simulink model "VOO_STATE"  (R2020a)
settings: Solver=FixedStepAuto  StartTime=0.0  StopTime=10.0  FixedStep=1e-3  RelTol=1e-3  EnableMultiTasking=on
undefined symbols (not defined in the file): D10, D12, D2, D5, D7, D9, PTA2, PTB9, PTC3, PTC4, PTD0, PTD3
libraries: frdmk64flib x8
settings Model: ExtModeTrigDuration=5  Creator=marry  LastModifiedBy=marry
settings OptimizationCC: EnhancedBackFolding=on  PassReuseOutputArgsAs=Individual arguments  ZeroExternalMemoryAtStartup=off  ZeroInternalMemoryAtStartup=off  MaxStackSize=64  OptimizeBlockOrder=speed  DifferentSizesBufferReuse=on  OptimizationCustomize=off  EfficientTunableParamExpr=on
settings DebuggingCC: ParameterTunabilityLossMsg=error
settings HardwareCC: ProdBitPerPointer=32  ProdBitPerSizeT=32  ProdBitPerPtrDiffT=32  ProdLargestAtomicInteger=Long  ProdLargestAtomicFloat=Double  ProdWordSize=32  ProdHWDeviceType=ARM Compatible->ARM Cortex
settings SFSimCC: MATLABDynamicMemAlloc=off
settings RTWCC: SystemTargetFile=ert.tlc  HardwareBoard=NXP FRDM-K64F  TemplateMakefile=ert_default_tmf  Toolchain=GNU Tools for ARM Embedded Processors
settings CodeAppCC: ForceParamTrailComments=on  IgnoreCustomStorageClasses=off  OperatorAnnotations=on  SimulinkDataObjDesc=on  SFDataObjDesc=on  InsertBlockDesc=on

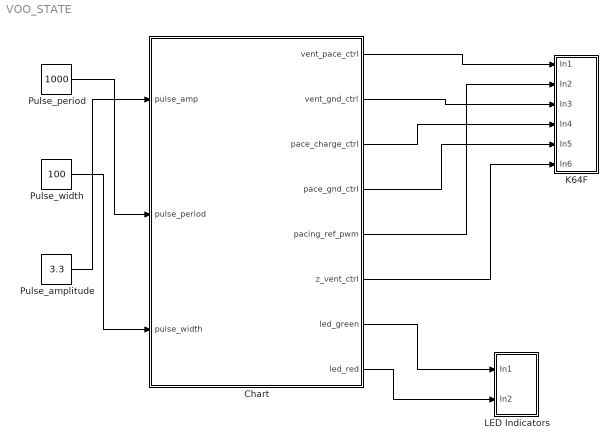
== system VOO_STATE ==
  Chart : Stateflow chart  TreatAsAtomicUnit=on
  K64F : Subsystem
  LED Indicators : Subsystem
  Pulse_amplitude : Constant  Value=3.3
  Pulse_period : Constant  Value=1000
  Pulse_width : Constant  Value=100
  wires:
  Chart/6(z_vent_ctrl) -> K64F/6(In6)
  Chart/4(pace_gnd_ctrl) -> K64F/5(In5)
  Chart/7(led_green) -> LED Indicators/1(In1)
  Chart/3(pace_charge_ctrl) -> K64F/4(In4)
  Chart/2(vent_gnd_ctrl) -> K64F/3(In3)
  Pulse_width/1 -> Chart/3(pulse_width)
  Chart/8(led_red) -> LED Indicators/2(In2)
  Pulse_amplitude/1 -> Chart/1(pulse_amp)
  Chart/1(vent_pace_ctrl) -> K64F/1(In1)
  Pulse_period/1 -> Chart/2(pulse_period)
  Chart/5(pacing_ref_pwm) -> K64F/2(In2)

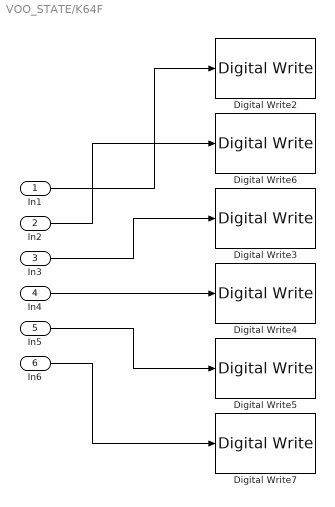
== system VOO_STATE/K64F ==
  In1 : Inport
  In2 : Inport  Port=2
  In3 : Inport  Port=3
  In4 : Inport  Port=4
  In5 : Inport  Port=5
  In6 : Inport  Port=6
  Digital Write2 : frdmk64flib/Digital Write  Whichpin=PTC4 (D9)
  Digital Write3 : frdmk64flib/Digital Write  Whichpin=PTD3 (D12)
  Digital Write4 : frdmk64flib/Digital Write  Whichpin=PTB9 (D2)
  Digital Write5 : frdmk64flib/Digital Write  Whichpin=PTD0 (D10)
  Digital Write6 : frdmk64flib/Digital Write  Whichpin=PTA2 (D5)
  Digital Write7 : frdmk64flib/Digital Write  Whichpin=PTC3 (D7)
  wires:
  In2/1 -> Digital Write6/1
  In1/1 -> Digital Write2/1
  In3/1 -> Digital Write3/1
  In4/1 -> Digital Write4/1
  In6/1 -> Digital Write7/1
  In5/1 -> Digital Write5/1

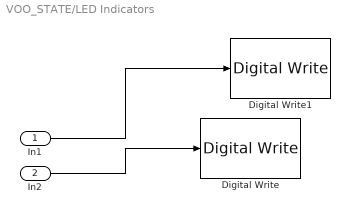
== system VOO_STATE/LED Indicators ==
  In1 : Inport
  In2 : Inport  Port=2
  Digital Write : frdmk64flib/Digital Write  Whichpin=RED_LED
  Digital Write1 : frdmk64flib/Digital Write  Whichpin=GREEN_LED
  wires:
  In1/1 -> Digital Write1/1
  In2/1 -> Digital Write/1

== stateflow chart VOO_STATE/Chart ==
  state AOO_Entry
    % Initial state when AOO is activated
    % Charging C22
    entry:
    vent_pace_ctrl = false;
    vent_gnd_ctrl = true;
    pace_charge_ctrl = true;
    pace_gnd_ctrl = true;
    pacing_ref_pwm = pulse_amp*20;
    z_vent_ctrl = 0;
    % LED indicator
    led_green = true;
    led_red = false;
  state AOO_Pace
    % Discharging current into the heart
    entry:
    pace_charge_ctrl = false;
    vent_gnd_ctrl = false;
    vent_pace_ctrl = true;
    % LED indicator
    led_green = false;
    led_red = true;
  state AOO_Charge
    % Charging C22 and C21 for cycles
    entry:
    vent_pace_ctrl = false;
    pace_charge_ctrl = true;
    vent_gnd_ctrl = true;
    % LED indicator
    led_green = true;
    led_red = false;
  (default) -> AOO_Entry
  AOO_Entry -> AOO_Pace : [after(pulse_period, msec)]
  AOO_Pace -> AOO_Charge : [after(pulse_width, msec)]
  AOO_Charge -> AOO_Pace : [after(pulse_period, msec)]
  data: pulse_amp input; pulse_period input; pulse_width input; vent_pace_ctrl output; vent_gnd_ctrl output; pace_charge_ctrl output; pace_gnd_ctrl output; pacing_ref_pwm output; z_vent_ctrl output; led_green output; led_red output
